simulink library "libc_control_pressure"  (R2015b)
settings: Solver=FixedStepDiscrete  StartTime=0.0  StopTime=Inf  FixedStep=0.004  RelTol=1e-3
PostLoadFcn:
  | , if any(exist('dsrtsu_mdlpostloadfcn', 'file') == [2, 3, 6]), try dsrtsu_mdlpostloadfcn('Execute', bdroot); catch fprintf('Error in PostLoadFcn (dsrtsu_mdlpostloadfcn) for model "%s":\n %s\n', bdroot, lasterr); end, end,
undefined symbols (not defined in the file or in its folder): CONST, den, DiscIntNeverNeededParam, num, p1i, tA
libraries: simulink x21, libc_parts_valves x17, libc_filters_diff x9, libbha_parts_bellows x4, libc_parts_tubes x2, PMC_lib x1
(part 2 of 2)

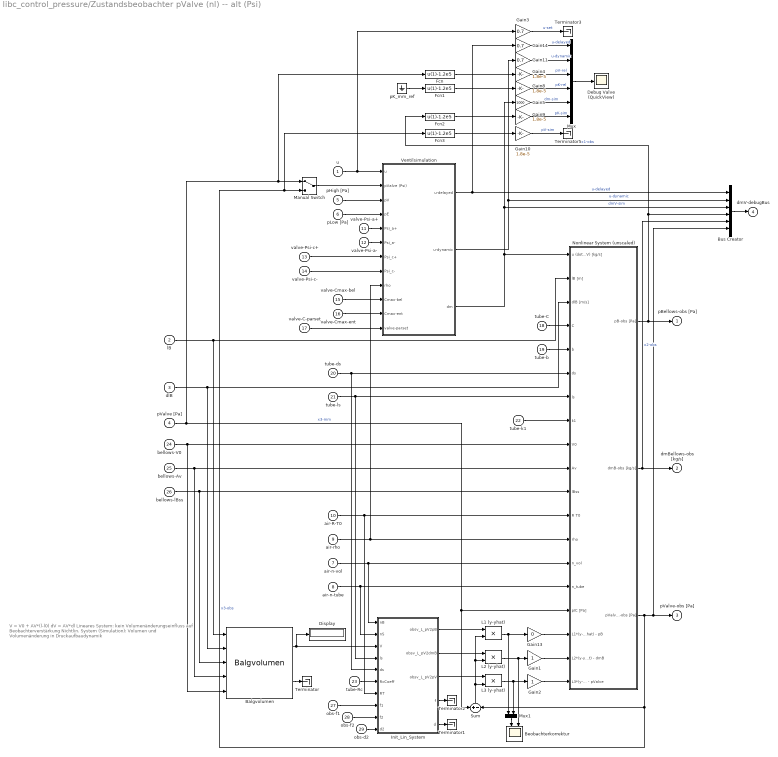
== system libc_control_pressure/Zustandsbeobachter pValve (nl) -- alt (Psi) ==
  note: V = V0 + AV*(l-l0)
      | dV = AV*dl
      |
      | Lineares System:
      | kein Volumenänderungseinfluss auf Beobachterverstärkung
      |
      | Nichtlin. System (Simulation):
      | Volumen und Volumenänderung in Druckaufbaudynamik
  u : Inport
  lB : Inport  Port=2
  dlB : Inport  Port=3
  pValve [Pa] : Inport  Port=4
  pHigh [Pa] : Inport  Port=5
  pLow [Pa] : Inport  Port=6
  air-n-vol : Inport  Port=7
  air-n-tube : Inport  Port=8
  air-rho : Inport  Port=9
  air-R-T0 : Inport  Port=10
  valve-Psi-a+ : Inport  Port=11
  valve-Psi-a- : Inport  Port=12
  valve-Psi-c+ : Inport  Port=13
  valve-Psi-c- : Inport  Port=14
  valve-Cmax-bel : Inport  Port=15
  valve-Cmax-ent : Inport  Port=16
  valve-C-parset : Inport  Port=17
  tube-C : Inport  Port=18
  tube-b : Inport  Port=19
  tube-ds : Inport  Port=20
  tube-ls : Inport  Port=21
  tube-k1 : Inport  Port=22
  tube-Rc : Inport  Port=23
  bellows-V0 : Inport  Port=24
  bellows-Av : Inport  Port=25
  bellows-lBss : Inport  Port=26
  obs-f1 : Inport  Port=27
  obs-f2 : Inport  Port=28
  obs-d2 : Inport  Port=29
  Balgvolumen : libbha_parts_bellows/Balgvolumen
  Beobachterkorrektur : Scope  NumInputPorts=2
  Bus Creator : BusCreator  Inputs=6
  Debug Valve (QuickView) : Scope
  Display : Display
  Fcn{,1..3} (4 alike) : Fcn  Expr=u(1)-1.2e5
  Gain1 : Gain
  Gain{4,8..10} (4 alike) : Gain  Gain=1.8e-5
  Gain11 : Gain  Gain=0.7
  Gain13 : Gain  Gain=0
  Gain14 : Gain  Gain=0.7
  Gain2 : Gain
  Gain3 : Gain  Gain=0.7
  Gain5 : Gain  Gain=1000
  Init_Lin_System : MATLAB Function  TreatAsAtomicUnit=on
  L1 (y-yhat) : Product
      settings: AttributesFormatString=sat: 0.1e5
  L2 (y-yhat) : Product
  L3 (y-yhat) : Product
  Manual Switch : ManualSwitch
  Mux : Mux  Inputs=6
  Mux1 : Mux  Inputs=2
  Nonlinear System (unscaled) : Subsystem
  Sum : Sum  Inputs=+|-
  Terminator{,1..3,5} (5 alike) : Terminator
  Ventilsimulation : Subsystem
  pK_mm_ref : Ground
  pBellows-obs [Pa] : Outport  PortDimensions=1
  dmBellows-obs [kg/s] : Outport  Port=2  PortDimensions=1
  pValve-obs [Pa] : Outport  Port=3  PortDimensions=1
  dmV-debugBus : Outport  Port=4
  wires:
  Gain14/1 -> Mux/1  "u-delayed"
  Ventilsimulation/2(u-dynamic) -> Gain11/1, Bus Creator/2  "u-dynamic"
  Gain13/1 -> Nonlinear System (unscaled)/17(L1*(y-yhat) - pB)
  Gain2/1 -> Nonlinear System (unscaled)/19(L3*(y-yhat) - pValve)
  Gain1/1 -> Nonlinear System (unscaled)/18(L2*(y-yhat) - dmB)
  Mux1/1 -> Beobachterkorrektur/1
  valve-Cmax-ent/1 -> Ventilsimulation/11(Cmax-ent)
  Gain11/1 -> Mux/2  "u-dynamic"
  Ventilsimulation/1(u-delayed) -> Gain14/1, Bus Creator/1  "u-delayed"
  Manual Switch/1 -> Ventilsimulation/2(pValve (Psi))
  Gain10/1 -> Terminator5/1  "pV-sim"
  Fcn3/1 -> Gain10/1
  Fcn2/1 -> Gain9/1
  Gain9/1 -> Mux/6  "pK-sim"
  Gain8/1 -> Mux/4  "pK-rel"
  Fcn1/1 -> Gain8/1
  pK_mm_ref/1 -> Fcn1/1
  Mux/1 -> Debug Valve (QuickView)/1
  Fcn/1 -> Gain4/1
  Gain5/1 -> Mux/5  "dm-sim"
  Gain4/1 -> Mux/3  "pV-rel"
  Gain3/1 -> Terminator3/1  "u-set"
  air-n-vol/1 -> Nonlinear System (unscaled)/14(n_vol), Init_Lin_System/1(nB)
  Ventilsimulation/3(dm) -> Nonlinear System (unscaled)/1(u (dotmV) [kg/s]), Gain5/1, Bus Creator/3  "dmV-sim"
  Init_Lin_System/4(f) -> Terminator2/1
  Init_Lin_System/5(d) -> Terminator1/1
  valve-Psi-c-/1 -> Ventilsimulation/8(Psi_c-)
  valve-Psi-c+/1 -> Ventilsimulation/7(Psi_c+)
  valve-Psi-a-/1 -> Ventilsimulation/6(Psi_a-)
  obs-f2/1 -> Init_Lin_System/9(f2)
  obs-d2/1 -> Init_Lin_System/10(d2)
  obs-f1/1 -> Init_Lin_System/8(f1)
  pLow [Pa]/1 -> Ventilsimulation/4(pE)
  pHigh [Pa]/1 -> Ventilsimulation/3(pV)
  valve-C-parset/1 -> Ventilsimulation/12(valve-parset)
  valve-Psi-a+/1 -> Ventilsimulation/5(Psi_a+)
  valve-Cmax-bel/1 -> Ventilsimulation/10(Cmax-bel)
  air-R-T0/1 -> Nonlinear System (unscaled)/12(R T0), Init_Lin_System/7(RT)
  air-rho/1 -> Ventilsimulation/9(rho), Nonlinear System (unscaled)/13(rho)
  u/1 -> Ventilsimulation/1(u), Gain3/1
  tube-Rc/1 -> Init_Lin_System/6(RcCoeff)
  bellows-Av/1 -> Nonlinear System (unscaled)/10(Av), Balgvolumen/4
  dlB/1 -> Nonlinear System (unscaled)/3(dlB [m/s]), Balgvolumen/2
  Balgvolumen/2 -> Terminator/1
  Balgvolumen/1 -> Init_Lin_System/3(V), Display/1
  tube-ls/1 -> Nonlinear System (unscaled)/7(ls), Init_Lin_System/4(ls)
  bellows-lBss/1 -> Nonlinear System (unscaled)/11(lBss), Balgvolumen/3
  bellows-V0/1 -> Nonlinear System (unscaled)/9(V0), Balgvolumen/5
  air-n-tube/1 -> Nonlinear System (unscaled)/15(n_tube), Init_Lin_System/2(nS)
  tube-k1/1 -> Nonlinear System (unscaled)/8(k1)
  lB/1 -> Nonlinear System (unscaled)/2(lB [m]), Balgvolumen/1
  tube-b/1 -> Nonlinear System (unscaled)/5(b)
  Init_Lin_System/1(obsv_L_pV2pB) -> L1 (y-yhat)/1
  Init_Lin_System/3(obsv_L_pV2pV) -> L3 (y-yhat)/1
  Init_Lin_System/2(obsv_L_pV2dmB) -> L2 (y-yhat)/1
  L3 (y-yhat)/1 -> Gain2/1, Mux1/2
  L2 (y-yhat)/1 -> Beobachterkorrektur/2, Gain1/1
  Nonlinear System (unscaled)/2(dmB-obs [kg/s]) -> dmBellows-obs [kg/s]/1, Bus Creator/5  "x2-obs"
  Nonlinear System (unscaled)/1(pB-obs [Pa]) -> pBellows-obs [Pa]/1, Bus Creator/4, Fcn2/1  "x1-obs"
  Nonlinear System (unscaled)/3(pValve-obs [Pa]) -> pValve-obs [Pa]/1, Bus Creator/6, Manual Switch/2, Fcn3/1, Sum/2  "x3-obs"
  Sum/1 -> L3 (y-yhat)/2, L2 (y-yhat)/2, L1 (y-yhat)/2
  L1 (y-yhat)/1 -> Gain13/1, Mux1/1
  pValve [Pa]/1 -> Manual Switch/1, Fcn/1, Nonlinear System (unscaled)/16(pIC [Pa]), Sum/1  "x3-mm"
  tube-C/1 -> Nonlinear System (unscaled)/4(C)
  tube-ds/1 -> Nonlinear System (unscaled)/6(ds), Init_Lin_System/5(ds)
  Bus Creator/1 -> dmV-debugBus/1

== system libc_control_pressure/Druckregler/Drucklinearsierung ==
  nu_in_PReg : Inport
  nu_in_Vorst : Inport  Port=2
  V : Inport  Port=3
  dV : Inport  Port=4
  p (E/A) : Inport  Port=5
  RT0 : Inport  Port=6
  nK : Inport  Port=7
  -Lf : Product  Inputs=*/**
  1/Lgx : Product  Inputs=//*
  mdot_soll : Product  Inputs=**
  nu-Lfx : Sum  Inputs=++|+
      settings: AttributesFormatString=|
      | früher ++-,
      | das ist aber falsch gewesen
  dm : Outport
  wires:
  p (E/A)/1 -> -Lf/4
  dV/1 -> -Lf/3
  -Lf/1 -> nu-Lfx/3
  mdot_soll/1 -> dm/1
  1/Lgx/1 -> mdot_soll/1
  nu-Lfx/1 -> mdot_soll/2
  nu_in_Vorst/1 -> nu-Lfx/2
  nu_in_PReg/1 -> nu-Lfx/1
  V/1 -> 1/Lgx/3, -Lf/2
  RT0/1 -> 1/Lgx/1
  nK/1 -> 1/Lgx/2, -Lf/1

== system libc_control_pressure/Druckregler/Folgeregler ==
  note: Vorsteuerung
  note: P-Regler
  p_soll : Inport
  dp_soll : Inport  Port=2
  p_ist : Inport  Port=3
  ctrl [ fgP enP enV ] : Inport  Port=4
  Demux : Demux  Outputs=3
  Product : Product
  Sw1 : Switch  Threshold=0.5
  Sw3 : Switch  Threshold=0.5
  null : Constant  Value=0
  null1 : Constant  Value=0
  omaga[rad/s] : Gain  Gain=2*pi
  reg_fehler : Sum  Inputs=+-
  e : Outport
  nu_P : Outport  Port=2
  nu_Vst : Outport  Port=3
  wires:
  Demux/1 -> omaga[rad/s]/1
  Product/1 -> Sw1/1
  null1/1 -> Sw1/3
  Demux/2 -> Sw1/2
  Demux/3 -> Sw3/2
  Sw1/1 -> nu_P/1
  Sw3/1 -> nu_Vst/1
  null/1 -> Sw3/3
  ctrl [ fgP enP enV ]/1 -> Demux/1
  dp_soll/1 -> Sw3/1
  reg_fehler/1 -> e/1, Product/1
  omaga[rad/s]/1 -> Product/2
  p_ist/1 -> reg_fehler/2
  p_soll/1 -> reg_fehler/1

== system libc_control_pressure/Ventilinvertierung FMText/Berechnung Ventilstellsignale mod-fav ==
  mp2_soll : Inport
  p2 : Inport  Port=2
  p1 : Inport  Port=3
  p0 : Inport  Port=4
  Ventilparam : Inport  Port=5  OutDataTypeStr=Bus: st_VentilParameter
  psi_min : Inport  Port=6
  kein_rueckstrom : Inport  Port=7
  BerechnungVentilstellsignale : Subsystem
      mask help: Umrechnung eines gewünschten Massenstroms in ein entsprechendes Ventilstellsignal.
  Bus Selector : BusSelector  OutputSignals=BP,BR
  Data Type Conversion : DataTypeConversion  OutDataTypeStr=double
  Product : Product
  Relational Operator : RelationalOperator  Operator=>  OutDataTypeStr=boolean
  Split_u : Subsystem
  Switch : Switch  Criteria=u2 > Threshold  Threshold=0.5
  Switch1 : Switch  Criteria=u2 > Threshold  Threshold=0.5
  Switch2 : Switch  Criteria=u2 > Threshold  Threshold=0.5
  inverse : Constant  Value=-1
  normal : Constant
  u : Outport
  wires:
  kein_rueckstrom/1 -> BerechnungVentilstellsignale/8(kein_rueckstrom)
  psi_min/1 -> BerechnungVentilstellsignale/7(psimin)
  Data Type Conversion/1 -> Switch/2, Switch1/2, Switch2/2
  Relational Operator/1 -> Data Type Conversion/1
  p0/1 -> Switch/3, Switch1/1, Relational Operator/2
  p1/1 -> Switch/1, Switch1/3, Relational Operator/1
  inverse/1 -> Switch2/3
  normal/1 -> Switch2/1
  Switch2/1 -> Product/1
  Product/1 -> Split_u/1(ut)
  BerechnungVentilstellsignale/1(ut) -> Product/2
  Switch1/1 -> BerechnungVentilstellsignale/4(p0_low)
  Switch/1 -> BerechnungVentilstellsignale/3(p1_high)
  Bus Selector/2 -> BerechnungVentilstellsignale/6(BR)  "<BR>"
  Bus Selector/1 -> BerechnungVentilstellsignale/5(BP)  "<BP>"
  Ventilparam/1 -> Bus Selector/1
  p2/1 -> BerechnungVentilstellsignale/2(p2_valve)
  mp2_soll/1 -> BerechnungVentilstellsignale/1(mp2_soll)
  Split_u/1(u) -> u/1

== system libc_control_pressure/Ventilinvertierung FMText/limit_p2 ==
  pV : Inport
  pH : Inport  Port=2
  pL : Inport  Port=3
  limit : Inport  Port=4
  Saturation Dynamic : simulink/Discontinuities/Saturation Dynamic  OutMin=[]  OutMax=[]  OutDataTypeStr=Inherit: Same as second input  OutDataType=fixdt(1, 16)  OutScaling=2^-10  DoSatur=off
  Sum : Sum  Inputs=|++
  Sum1 : Sum  Inputs=|+-
  dP [pA] : Constant  Value=0.1
  sw_p2s : Switch  Criteria=u2 > Threshold  Threshold=0.5
  pVlim : Outport
  wires:
  sw_p2s/1 -> pVlim/1
  pV/1 -> Saturation Dynamic/2, sw_p2s/3
  Saturation Dynamic/1 -> sw_p2s/1
  limit/1 -> sw_p2s/2
  Sum/1 -> Saturation Dynamic/3
  pL/1 -> Sum/1
  pH/1 -> Sum1/1
  Sum1/1 -> Saturation Dynamic/1
  dP [pA]/1 -> Sum/2, Sum1/2

== system libc_control_pressure/Ventilinvertierung FMText_simple/Berechnung Ventilstellsignale mod-fav ==
  mp2_soll : Inport
  p2 : Inport  Port=2
  p1 : Inport  Port=3
  p0 : Inport  Port=4
  Ventilparam : Inport  Port=5  OutDataTypeStr=Bus: st_VentilParameter
  psi_min : Inport  Port=6
  kein_rueckstrom : Inport  Port=7
  BerechnungVentilstellsignale : Subsystem
      mask help: Umrechnung eines gewünschten Massenstroms in ein entsprechendes Ventilstellsignal.
  Bus Selector : BusSelector  OutputSignals=BP,BR
  Data Type Conversion : DataTypeConversion  OutDataTypeStr=double
  Product : Product
  Relational Operator : RelationalOperator  Operator=>  OutDataTypeStr=boolean
  Split_u : Subsystem
  Switch : Switch  Criteria=u2 > Threshold  Threshold=0.5
  Switch1 : Switch  Criteria=u2 > Threshold  Threshold=0.5
  Switch2 : Switch  Criteria=u2 > Threshold  Threshold=0.5
  inverse : Constant  Value=-1
  normal : Constant
  u : Outport
  wires:
  Split_u/1(u) -> u/1
  mp2_soll/1 -> BerechnungVentilstellsignale/1(mp2_soll)
  p2/1 -> BerechnungVentilstellsignale/2(p2_valve)
  Ventilparam/1 -> Bus Selector/1
  Bus Selector/1 -> BerechnungVentilstellsignale/5(BP)  "<BP>"
  Bus Selector/2 -> BerechnungVentilstellsignale/6(BR)  "<BR>"
  Switch/1 -> BerechnungVentilstellsignale/3(p1_high)
  Switch1/1 -> BerechnungVentilstellsignale/4(p0_low)
  BerechnungVentilstellsignale/1(ut) -> Product/2
  Product/1 -> Split_u/1(ut)
  Switch2/1 -> Product/1
  normal/1 -> Switch2/1
  inverse/1 -> Switch2/3
  p1/1 -> Relational Operator/1, Switch1/3, Switch/1
  p0/1 -> Relational Operator/2, Switch1/1, Switch/3
  Relational Operator/1 -> Data Type Conversion/1
  Data Type Conversion/1 -> Switch2/2, Switch1/2, Switch/2
  psi_min/1 -> BerechnungVentilstellsignale/7(psimin)
  kein_rueckstrom/1 -> BerechnungVentilstellsignale/8(kein_rueckstrom)

== system libc_control_pressure/Ventilinvertierung FMText_simple/limit_p2 ==
  pV : Inport
  pH : Inport  Port=2
  pL : Inport  Port=3
  limit : Inport  Port=4
  Saturation Dynamic : simulink/Discontinuities/Saturation Dynamic  OutMin=[]  OutMax=[]  OutDataTypeStr=Inherit: Same as second input  OutDataType=fixdt(1, 16)  OutScaling=2^-10  DoSatur=off
  Sum : Sum  Inputs=|++
  Sum1 : Sum  Inputs=|+-
  dP [pA] : Constant  Value=0.1
  sw_p2s : Switch  Criteria=u2 > Threshold  Threshold=0.5
  pVlim : Outport
  wires:
  dP [pA]/1 -> Sum1/2, Sum/2
  Sum1/1 -> Saturation Dynamic/1
  pH/1 -> Sum1/1
  pL/1 -> Sum/1
  Sum/1 -> Saturation Dynamic/3
  limit/1 -> sw_p2s/2
  Saturation Dynamic/1 -> sw_p2s/1
  pV/1 -> sw_p2s/3, Saturation Dynamic/2
  sw_p2s/1 -> pVlim/1

== system libc_control_pressure/Ventilinvertierung MPYE/Psi Param ==
  b : Inport
  b-auto : MATLAB Function  TreatAsAtomicUnit=on
  a1 : Outport
  a2 : Outport  Port=2
  c0 : Outport  Port=3
  wires:
  b-auto/2(a2) -> a2/1
  b-auto/3(c0) -> c0/1
  b-auto/1(a1) -> a1/1
  b/1 -> b-auto/1(b)

== system libc_control_pressure/Zustandsbeobachter pValve (nl)/Nonlinear System (unscaled) ==
  u (dotmV) [kg/s] : Inport
  lB [m] : Inport  Port=2
  dlB [m/s] : Inport  Port=3
  C : Inport  Port=4
  b : Inport  Port=5
  ds : Inport  Port=6
  ls : Inport  Port=7
  k1 : Inport  Port=8
  V0 : Inport  Port=9
  Av : Inport  Port=10
  lBss : Inport  Port=11
  R T0 : Inport  Port=12
  rho : Inport  Port=13
  n_vol : Inport  Port=14
  n_tube : Inport  Port=15
  pIC [Pa] : Inport  Port=16
  L1*(y-yhat) - pB : Inport  Port=17
  L2*(y-yhat) - dmB : Inport  Port=18
  L3*(y-yhat) - pValve : Inport  Port=19
  Druckaufbau Balg : Subsystem
  Schlauchmodell 2. Ordnung (allg) : libc_parts_tubes/Schlauchmodell 2. Ordnung (allg)
  no_mf : Constant  Value=0
  pB-obs [Pa] : Outport
  dmB-obs [kg/s] : Outport  Port=2
  pValve-obs [Pa] : Outport  Port=3
  wires:
  n_vol/1 -> Druckaufbau Balg/5(n)
  Av/1 -> Druckaufbau Balg/8(Av)
  dlB [m/s]/1 -> Druckaufbau Balg/3(dlb [m/s])
  lBss/1 -> Druckaufbau Balg/7(lBss)
  V0/1 -> Druckaufbau Balg/9(V0)
  lB [m]/1 -> Druckaufbau Balg/2(lb [m])
  rho/1 -> Schlauchmodell 2. Ordnung (allg)/11
  R T0/1 -> Schlauchmodell 2. Ordnung (allg)/10, Druckaufbau Balg/6(RT0)
  b/1 -> Schlauchmodell 2. Ordnung (allg)/6
  u (dotmV) [kg/s]/1 -> Schlauchmodell 2. Ordnung (allg)/2
  pIC [Pa]/1 -> Druckaufbau Balg/1(pB_0), Schlauchmodell 2. Ordnung (allg)/3
  L3*(y-yhat) - pValve/1 -> Schlauchmodell 2. Ordnung (allg)/13
  L2*(y-yhat) - dmB/1 -> Schlauchmodell 2. Ordnung (allg)/14
  L1*(y-yhat) - pB/1 -> Druckaufbau Balg/10(L_pB)
  Schlauchmodell 2. Ordnung (allg)/2 -> pValve-obs [Pa]/1
  Druckaufbau Balg/1(p [Pa]) -> pB-obs [Pa]/1, Schlauchmodell 2. Ordnung (allg)/1
  Schlauchmodell 2. Ordnung (allg)/1 -> Druckaufbau Balg/4(mp [kg/s]), dmB-obs [kg/s]/1
  no_mf/1 -> Schlauchmodell 2. Ordnung (allg)/4
  C/1 -> Schlauchmodell 2. Ordnung (allg)/5
  ds/1 -> Schlauchmodell 2. Ordnung (allg)/7
  ls/1 -> Schlauchmodell 2. Ordnung (allg)/8
  n_tube/1 -> Schlauchmodell 2. Ordnung (allg)/12
  k1/1 -> Schlauchmodell 2. Ordnung (allg)/9

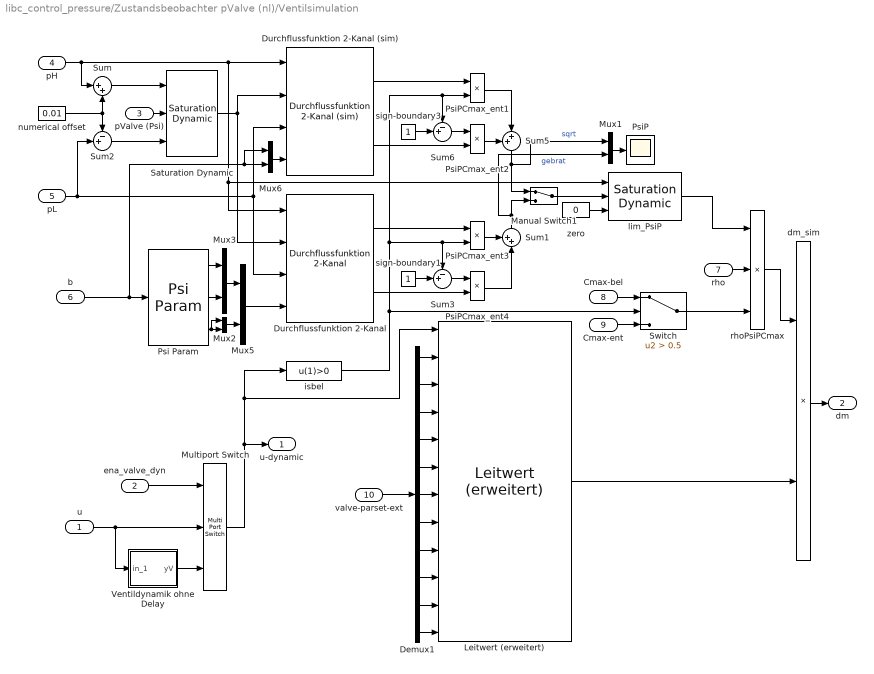
== system libc_control_pressure/Zustandsbeobachter pValve (nl)/Ventilsimulation ==
  u : Inport
  ena_valve_dyn : Inport  Port=2
  pValve (Psi) : Inport  Port=3
  pH : Inport  Port=4
  pL : Inport  Port=5
  b : Inport  Port=6
  rho : Inport  Port=7
  Cmax-bel : Inport  Port=8
  Cmax-ent : Inport  Port=9
  valve-parset-ext : Inport  Port=10
  Demux1 : Demux  Outputs=11
  Durchflussfunktion 2-Kanal : libc_parts_valves/Durchflussfunktion 2-Kanal
      settings: AttributesFormatString=gebrochenrational
  Durchflussfunktion 2-Kanal (sim) : libc_parts_valves/Durchflussfunktion 2-Kanal (sim)
      settings: AttributesFormatString=|
      | Wurzelfunktion
      | (nicht geeignet für Ventilinvertierung)
  Leitwert (erweitert) : libc_parts_valves/Leitwert (erweitert)  invertcomp=off
      settings: AttributesFormatString=|
      | inv: Cn --> u (on)
      | hin: u --> Cn (off)
      | Invertiert: %<invertcomp>
  Manual Switch1 : ManualSwitch
  Multiport Switch : MultiPortSwitch  DataPortOrder=Zero-based contiguous  Inputs=2
  Mux{1..3,5..6} (5 alike) : Mux  Inputs=2
  Psi Param : libc_parts_valves/Psi Param
      settings: AttributesFormatString=sqrt -> geb-rat
  PsiP : Scope
  PsiPCmax_ent{1..4} (4 alike) : Product
  Saturation Dynamic : simulink/Discontinuities/Saturation Dynamic  OutMin=[]  OutMax=[]  OutDataTypeStr=Inherit: Same as second input  OutDataType=fixdt(1, 16)  OutScaling=2^-10  DoSatur=off
  Sum : Sum  Inputs=|++
  Sum1 : Sum  Inputs=++|
  Sum2 : Sum  Inputs=-+|
  Sum3 : Sum  Inputs=-+|
  Sum5 : Sum  Inputs=++|
  Sum6 : Sum  Inputs=-+|
  Switch : Switch  Criteria=u2 > Threshold  Threshold=0.5
  Ventildynamik ohne Delay : Subsystem  mask(Ventilverzoegerung){wv=200*2*pi, dv=0.6, grenze=0.3, offset=0}
      mask prompts: wv "Eigenfreqenz"; dv "Daempfung"; grenze "Begrenzung"
      mask help: System 2. Ord. mit Begrenzung
      mask init:
      | [num,den]=ord2(wv,dv); t=0:0.5/wv:15/wv; u=0*t+1; u(1)=0;  y=lsim(num,den,u,t);
      mask Display: plot([0:0.1:1],[0 0.05 0.5 0.9 1.0 0.93 0.93 0.97 0.95 0.95 0.95]);
  dm_sim : Product  Inputs=**
  isbel : Fcn  Expr=u(1)>0
  lim_PsiP : simulink/Discontinuities/Saturation Dynamic  OutMin=[]  OutMax=[]  OutDataTypeStr=Inherit: Same as second input  OutDataType=fixdt(1, 16)  OutScaling=2^-10  DoSatur=off
      settings: AttributesFormatString=|
      | Unterer Schranke
      | im Entlüften nicht
      | pE sondern 0
  numerical offset : Constant  Value=0.01
  rhoPsiPCmax : Product  Inputs=***
  sign-boundary1 : Constant
  sign-boundary3 : Constant
  zero : Constant  Value=0
  u-dynamic : Outport
  dm : Outport  Port=2
  wires:
  dm_sim/1 -> dm/1
  Leitwert (erweitert)/1 -> dm_sim/2
  Demux1/1 -> Leitwert (erweitert)/2
  Demux1/2 -> Leitwert (erweitert)/3
  Demux1/5 -> Leitwert (erweitert)/6
  Demux1/6 -> Leitwert (erweitert)/7
  Demux1/3 -> Leitwert (erweitert)/4
  Demux1/4 -> Leitwert (erweitert)/5
  Demux1/7 -> Leitwert (erweitert)/8
  u/1 -> Multiport Switch/2, Ventildynamik ohne Delay/1(in_1)
  Multiport Switch/1 -> Leitwert (erweitert)/1, isbel/1, u-dynamic/1
  valve-parset-ext/1 -> Demux1/1
  Sum2/1 -> Saturation Dynamic/3
  numerical offset/1 -> Sum2/1, Sum/2
  pL/1 -> Sum2/2, Durchflussfunktion 2-Kanal (sim)/3, Durchflussfunktion 2-Kanal/3
  rhoPsiPCmax/1 -> dm_sim/1
  Saturation Dynamic/1 -> Durchflussfunktion 2-Kanal (sim)/2, Durchflussfunktion 2-Kanal/2
  pValve (Psi)/1 -> Saturation Dynamic/2
  lim_PsiP/1 -> rhoPsiPCmax/1
  Sum/1 -> Saturation Dynamic/1
  pH/1 -> Sum/1, Durchflussfunktion 2-Kanal (sim)/1, lim_PsiP/1, Durchflussfunktion 2-Kanal/1
  rho/1 -> rhoPsiPCmax/2
  Cmax-bel/1 -> Switch/1
  Ventildynamik ohne Delay/1(yV) -> Multiport Switch/3
  Switch/1 -> rhoPsiPCmax/3
  Cmax-ent/1 -> Switch/3
  zero/1 -> lim_PsiP/3
  ena_valve_dyn/1 -> Multiport Switch/1
  Demux1/9 -> Leitwert (erweitert)/10
  Demux1/10 -> Leitwert (erweitert)/11
  Demux1/8 -> Leitwert (erweitert)/9
  Demux1/11 -> Leitwert (erweitert)/12
  Mux1/1 -> PsiP/1
  Manual Switch1/1 -> lim_PsiP/2
  isbel/1 -> Switch/2, Sum3/1, PsiPCmax_ent3/2, Sum6/1, PsiPCmax_ent1/2
  b/1 -> Mux6/1, Mux6/2, Psi Param/1
  Mux5/1 -> Durchflussfunktion 2-Kanal/4
  Mux6/1 -> Durchflussfunktion 2-Kanal (sim)/4
  PsiPCmax_ent1/1 -> Sum5/2
  Durchflussfunktion 2-Kanal (sim)/1 -> PsiPCmax_ent1/1
  Durchflussfunktion 2-Kanal (sim)/2 -> PsiPCmax_ent2/2
  Sum6/1 -> PsiPCmax_ent2/1
  sign-boundary3/1 -> Sum6/2
  Durchflussfunktion 2-Kanal/1 -> PsiPCmax_ent3/1
  Durchflussfunktion 2-Kanal/2 -> PsiPCmax_ent4/2
  Sum3/1 -> PsiPCmax_ent4/1
  sign-boundary1/1 -> Sum3/2
  PsiPCmax_ent2/1 -> Sum5/1
  PsiPCmax_ent3/1 -> Sum1/1
  PsiPCmax_ent4/1 -> Sum1/2
  Sum1/1 -> Mux1/2, Manual Switch1/2  "gebrat"
  Sum5/1 -> Mux1/1, Manual Switch1/1  "sqrt"
  Psi Param/1 -> Mux3/1
  Psi Param/2 -> Mux3/2
  Psi Param/3 -> Mux2/1, Mux2/2
  Mux2/1 -> Mux5/2
  Mux3/1 -> Mux5/1

== system libc_control_pressure/Zustandsbeobachter pValve (nl) -- alt (Psi)/Nonlinear System (unscaled) ==
  u (dotmV) [kg/s] : Inport
  lB [m] : Inport  Port=2
  dlB [m/s] : Inport  Port=3
  C : Inport  Port=4
  b : Inport  Port=5
  ds : Inport  Port=6
  ls : Inport  Port=7
  k1 : Inport  Port=8
  V0 : Inport  Port=9
  Av : Inport  Port=10
  lBss : Inport  Port=11
  R T0 : Inport  Port=12
  rho : Inport  Port=13
  n_vol : Inport  Port=14
  n_tube : Inport  Port=15
  pIC [Pa] : Inport  Port=16
  L1*(y-yhat) - pB : Inport  Port=17
  L2*(y-yhat) - dmB : Inport  Port=18
  L3*(y-yhat) - pValve : Inport  Port=19
  Druckaufbau Balg : Subsystem
  Schlauchmodell 2. Ordnung (allg) : libc_parts_tubes/Schlauchmodell 2. Ordnung (allg)
  no_mf : Constant  Value=0
  pB-obs [Pa] : Outport
  dmB-obs [kg/s] : Outport  Port=2
  pValve-obs [Pa] : Outport  Port=3
  wires:
  n_vol/1 -> Druckaufbau Balg/5(n)
  Av/1 -> Druckaufbau Balg/8(Av)
  dlB [m/s]/1 -> Druckaufbau Balg/3(dlb [m/s])
  lBss/1 -> Druckaufbau Balg/7(lBss)
  V0/1 -> Druckaufbau Balg/9(V0)
  lB [m]/1 -> Druckaufbau Balg/2(lb [m])
  rho/1 -> Schlauchmodell 2. Ordnung (allg)/11
  R T0/1 -> Schlauchmodell 2. Ordnung (allg)/10, Druckaufbau Balg/6(RT0)
  b/1 -> Schlauchmodell 2. Ordnung (allg)/6
  u (dotmV) [kg/s]/1 -> Schlauchmodell 2. Ordnung (allg)/2
  pIC [Pa]/1 -> Druckaufbau Balg/1(pB_0), Schlauchmodell 2. Ordnung (allg)/3
  L3*(y-yhat) - pValve/1 -> Schlauchmodell 2. Ordnung (allg)/13
  L2*(y-yhat) - dmB/1 -> Schlauchmodell 2. Ordnung (allg)/14
  L1*(y-yhat) - pB/1 -> Druckaufbau Balg/10(L_pB)
  Schlauchmodell 2. Ordnung (allg)/2 -> pValve-obs [Pa]/1
  Druckaufbau Balg/1(p [Pa]) -> pB-obs [Pa]/1, Schlauchmodell 2. Ordnung (allg)/1
  Schlauchmodell 2. Ordnung (allg)/1 -> Druckaufbau Balg/4(mp [kg/s]), dmB-obs [kg/s]/1
  no_mf/1 -> Schlauchmodell 2. Ordnung (allg)/4
  C/1 -> Schlauchmodell 2. Ordnung (allg)/5
  ds/1 -> Schlauchmodell 2. Ordnung (allg)/7
  ls/1 -> Schlauchmodell 2. Ordnung (allg)/8
  n_tube/1 -> Schlauchmodell 2. Ordnung (allg)/12
  k1/1 -> Schlauchmodell 2. Ordnung (allg)/9

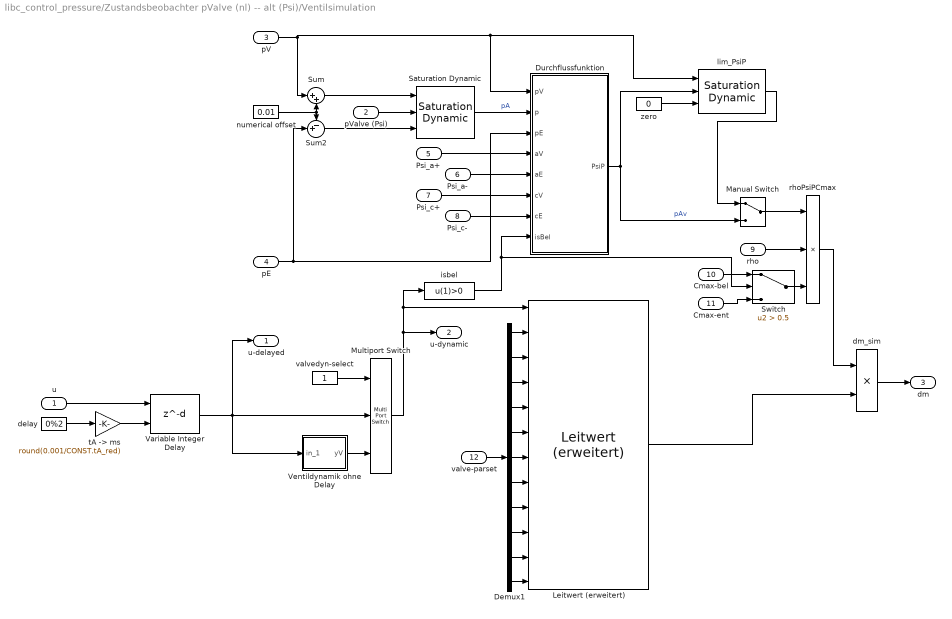
== system libc_control_pressure/Zustandsbeobachter pValve (nl) -- alt (Psi)/Ventilsimulation ==
  u : Inport
  pValve (Psi) : Inport  Port=2
  pV : Inport  Port=3
  pE : Inport  Port=4
  Psi_a+ : Inport  Port=5
  Psi_a- : Inport  Port=6
  Psi_c+ : Inport  Port=7
  Psi_c- : Inport  Port=8
  rho : Inport  Port=9
  Cmax-bel : Inport  Port=10
  Cmax-ent : Inport  Port=11
  valve-parset : Inport  Port=12
  Demux1 : Demux  Outputs=11
  Durchflussfunktion : MATLAB Function  TreatAsAtomicUnit=on
      settings: AttributesFormatString=saturated
  Leitwert (erweitert) : libc_parts_valves/Leitwert (erweitert)  invertcomp=off
      settings: AttributesFormatString=|
      | inv: Cn --> u (on)
      | hin: u --> Cn (off)
      | Invertiert: %<invertcomp>
  Manual Switch : ManualSwitch
  Multiport Switch : MultiPortSwitch  DataPortOrder=Zero-based contiguous  Inputs=2
  Saturation Dynamic : simulink/Discontinuities/Saturation Dynamic  OutMin=[]  OutMax=[]  OutDataTypeStr=Inherit: Same as second input  OutDataType=fixdt(1, 16)  OutScaling=2^-10  DoSatur=off
  Sum : Sum  Inputs=|++
  Sum2 : Sum  Inputs=-+|
  Switch : Switch  Criteria=u2 > Threshold  Threshold=0.5
  Variable Integer Delay : Delay  DelayLengthSource=Input port  DelayLength=0
      settings: AttributesFormatString=max delay %<DelayLengthUpperLimit>  InputPortMap=u0,p1
  Ventildynamik ohne Delay : Subsystem  mask(Ventilverzoegerung){wv=200*2*pi, dv=0.6, grenze=0.3, offset=0}
      mask prompts: wv "Eigenfreqenz"; dv "Daempfung"; grenze "Begrenzung"
      mask help: System 2. Ord. mit Begrenzung
      mask init:
      | [num,den]=ord2(wv,dv); t=0:0.5/wv:15/wv; u=0*t+1; u(1)=0;  y=lsim(num,den,u,t);
      mask Display: plot([0:0.1:1],[0 0.05 0.5 0.9 1.0 0.93 0.93 0.97 0.95 0.95 0.95]);
  delay : Constant  Value=0%2
      settings: AttributesFormatString=[ms] tA = 0.001
  dm_sim : Product  Inputs=**
  isbel : Fcn  Expr=u(1)>0
  lim_PsiP : simulink/Discontinuities/Saturation Dynamic  OutMin=[]  OutMax=[]  OutDataTypeStr=Inherit: Same as second input  OutDataType=fixdt(1, 16)  OutScaling=2^-10  DoSatur=off
      settings: AttributesFormatString=Unterer Schranke im Entlüften nicht pE sondern 0
  numerical offset : Constant  Value=0.01
  rhoPsiPCmax : Product  Inputs=***
  "tA -> ms" : Gain  Gain=round(0.001/CONST.tA_red)
  valvedyn-select : Constant
  zero : Constant  Value=0
  u-delayed : Outport
  u-dynamic : Outport  Port=2
  dm : Outport  Port=3
  wires:
  Demux1/11 -> Leitwert (erweitert)/12
  Demux1/10 -> Leitwert (erweitert)/11
  Demux1/9 -> Leitwert (erweitert)/10
  Demux1/8 -> Leitwert (erweitert)/9
  zero/1 -> lim_PsiP/3
  Cmax-ent/1 -> Switch/3
  Switch/1 -> rhoPsiPCmax/3
  "tA -> ms"/1 -> Variable Integer Delay/2
  delay/1 -> "tA -> ms"/1
  u/1 -> Variable Integer Delay/1
  valvedyn-select/1 -> Multiport Switch/1
  Ventildynamik ohne Delay/1(yV) -> Multiport Switch/3
  Psi_c-/1 -> Durchflussfunktion/7(cE)
  Psi_c+/1 -> Durchflussfunktion/6(cV)
  Psi_a-/1 -> Durchflussfunktion/5(aE)
  Cmax-bel/1 -> Switch/1
  rho/1 -> rhoPsiPCmax/2
  pV/1 -> lim_PsiP/1, Durchflussfunktion/1(pV), Sum/1
  Sum/1 -> Saturation Dynamic/1
  pValve (Psi)/1 -> Saturation Dynamic/2
  Saturation Dynamic/1 -> Durchflussfunktion/2(p)  "pA"
  Durchflussfunktion/1(PsiP) -> Manual Switch/2, lim_PsiP/2  "pAv"
  rhoPsiPCmax/1 -> dm_sim/1
  pE/1 -> Sum2/2, Durchflussfunktion/3(pE)
  numerical offset/1 -> Sum2/1, Sum/2
  Sum2/1 -> Saturation Dynamic/3
  Psi_a+/1 -> Durchflussfunktion/4(aV)
  valve-parset/1 -> Demux1/1
  Multiport Switch/1 -> isbel/1, Leitwert (erweitert)/1, u-dynamic/1
  Variable Integer Delay/1 -> Ventildynamik ohne Delay/1(in_1), Multiport Switch/2, u-delayed/1
  Demux1/7 -> Leitwert (erweitert)/8
  Demux1/4 -> Leitwert (erweitert)/5
  Demux1/3 -> Leitwert (erweitert)/4
  Demux1/6 -> Leitwert (erweitert)/7
  Demux1/5 -> Leitwert (erweitert)/6
  Demux1/2 -> Leitwert (erweitert)/3
  Demux1/1 -> Leitwert (erweitert)/2
  isbel/1 -> Durchflussfunktion/8(isBel), Switch/2
  Leitwert (erweitert)/1 -> dm_sim/2
  dm_sim/1 -> dm/1
  Manual Switch/1 -> rhoPsiPCmax/1
  lim_PsiP/1 -> Manual Switch/1

== system libc_control_pressure/Ventilinvertierung FMText/Berechnung Ventilstellsignale mod-fav/BerechnungVentilstellsignale ==
  mp2_soll : Inport
  p2_valve : Inport  Port=2
  p1_high : Inport  Port=3
  p0_low : Inport  Port=4
  BP : Inport  Port=5  OutDataTypeStr=Bus: st_Booster
  BR : Inport  Port=6  OutDataTypeStr=Bus: st_Booster
  psimin : Inport  Port=7
  kein_rueckstrom : Inport  Port=8
  Bus Selector : BusSelector  OutputSignals=C_max,b_max,b_min
  Bus Selector1 : BusSelector  OutputSignals=C_max,b_max,b_min
  Memory : Memory  InheritSampleTime=on
  Umrechnung Massenstrom in Ventilstellsignale : MATLAB Function
  ut : Outport
  wires:
  kein_rueckstrom/1 -> Umrechnung Massenstrom in Ventilstellsignale/12(kein_rueckstrom)
  psimin/1 -> Umrechnung Massenstrom in Ventilstellsignale/11(psimin)
  BR/1 -> Bus Selector1/1
  Bus Selector1/3 -> Umrechnung Massenstrom in Ventilstellsignale/10(bmin_ent)  "<b_min>"
  Bus Selector1/1 -> Umrechnung Massenstrom in Ventilstellsignale/8(C_ent)  "<C_max>"
  Bus Selector1/2 -> Umrechnung Massenstrom in Ventilstellsignale/9(b_ent)  "<b_max>"
  Bus Selector/2 -> Umrechnung Massenstrom in Ventilstellsignale/6(b_bel)  "<b_max>"
  Bus Selector/3 -> Umrechnung Massenstrom in Ventilstellsignale/7(bmin_bel)  "<b_min>"
  Bus Selector/1 -> Umrechnung Massenstrom in Ventilstellsignale/5(C_bel)  "<C_max>"
  BP/1 -> Bus Selector/1
  p1_high/1 -> Umrechnung Massenstrom in Ventilstellsignale/3(p1)
  p0_low/1 -> Umrechnung Massenstrom in Ventilstellsignale/4(p0)
  p2_valve/1 -> Umrechnung Massenstrom in Ventilstellsignale/2(p2)
  mp2_soll/1 -> Umrechnung Massenstrom in Ventilstellsignale/1(mp2)
  Memory/1 -> Umrechnung Massenstrom in Ventilstellsignale/13(ulast)
  Umrechnung Massenstrom in Ventilstellsignale/1(ut) -> Memory/1, ut/1

== system libc_control_pressure/Ventilinvertierung FMText/Berechnung Ventilstellsignale mod-fav/Split_u ==
  ut : Inport
  Gain : Gain  Gain=-1
  Mux : Mux  Inputs=2
  Saturation : Saturate  UpperLimit=1  LowerLimit=0
  Saturation1 : Saturate  UpperLimit=1  LowerLimit=0
  u : Outport
  wires:
  Saturation1/1 -> Mux/2
  Saturation/1 -> Mux/1
  Mux/1 -> u/1
  ut/1 -> Saturation/1, Gain/1
  Gain/1 -> Saturation1/1

== system libc_control_pressure/Ventilinvertierung FMText_simple/Berechnung Ventilstellsignale mod-fav/BerechnungVentilstellsignale ==
  mp2_soll : Inport
  p2_valve : Inport  Port=2
  p1_high : Inport  Port=3
  p0_low : Inport  Port=4
  BP : Inport  Port=5  OutDataTypeStr=Bus: st_Booster
  BR : Inport  Port=6  OutDataTypeStr=Bus: st_Booster
  psimin : Inport  Port=7
  kein_rueckstrom : Inport  Port=8
  Bus Selector : BusSelector  OutputSignals=C_max,b_max,b_min
  Bus Selector1 : BusSelector  OutputSignals=C_max,b_max,b_min
  Memory : Memory  InheritSampleTime=on
  Umrechnung Massenstrom in Ventilstellsignale : MATLAB Function
  ut : Outport
  wires:
  Umrechnung Massenstrom in Ventilstellsignale/1(ut) -> ut/1, Memory/1
  Memory/1 -> Umrechnung Massenstrom in Ventilstellsignale/13(ulast)
  mp2_soll/1 -> Umrechnung Massenstrom in Ventilstellsignale/1(mp2)
  p2_valve/1 -> Umrechnung Massenstrom in Ventilstellsignale/2(p2)
  p0_low/1 -> Umrechnung Massenstrom in Ventilstellsignale/4(p0)
  p1_high/1 -> Umrechnung Massenstrom in Ventilstellsignale/3(p1)
  BP/1 -> Bus Selector/1
  Bus Selector/1 -> Umrechnung Massenstrom in Ventilstellsignale/5(C_bel)  "<C_max>"
  Bus Selector/3 -> Umrechnung Massenstrom in Ventilstellsignale/7(bmin_bel)  "<b_min>"
  Bus Selector/2 -> Umrechnung Massenstrom in Ventilstellsignale/6(b_bel)  "<b_max>"
  Bus Selector1/2 -> Umrechnung Massenstrom in Ventilstellsignale/9(b_ent)  "<b_max>"
  Bus Selector1/1 -> Umrechnung Massenstrom in Ventilstellsignale/8(C_ent)  "<C_max>"
  Bus Selector1/3 -> Umrechnung Massenstrom in Ventilstellsignale/10(bmin_ent)  "<b_min>"
  BR/1 -> Bus Selector1/1
  psimin/1 -> Umrechnung Massenstrom in Ventilstellsignale/11(psimin)
  kein_rueckstrom/1 -> Umrechnung Massenstrom in Ventilstellsignale/12(kein_rueckstrom)

== system libc_control_pressure/Ventilinvertierung FMText_simple/Berechnung Ventilstellsignale mod-fav/Split_u ==
  ut : Inport
  Gain : Gain  Gain=-1
  Mux : Mux  Inputs=2
  Saturation : Saturate  UpperLimit=1  LowerLimit=0
  Saturation1 : Saturate  UpperLimit=1  LowerLimit=0
  u : Outport
  wires:
  Gain/1 -> Saturation1/1
  ut/1 -> Gain/1, Saturation/1
  Mux/1 -> u/1
  Saturation/1 -> Mux/1
  Saturation1/1 -> Mux/2

== system libc_control_pressure/Zustandsbeobachter pValve (nl)/Nonlinear System (unscaled)/Druckaufbau Balg ==
  pB_0 : Inport
  lb [m] : Inport  Port=2
  dlb [m/s] : Inport  Port=3
  mp [kg/s] : Inport  Port=4
  n : Inport  Port=5
  RT0 : Inport  Port=6
  lBss : Inport  Port=7
  Av : Inport  Port=8
  V0 : Inport  Port=9
  L_pB : Inport  Port=10
  Discrete-Time Integrator : DiscreteIntegrator  InitialConditionSource=external  InitialCondition=p1i  SampleTime=-1  ICPrevOutput=DiscIntNeverNeededParam  ICPrevScaledInput=DiscIntNeverNeededParam
  Druckdynamik (allg) : libbha_parts_bellows/Druckdynamik (allg)
  Sum1 : Sum  Inputs=|++
  p [Pa] : Outport  InitialOutput=0
  wires:
  V0/1 -> Druckdynamik (allg)/7
  Av/1 -> Druckdynamik (allg)/5
  lBss/1 -> Druckdynamik (allg)/6
  RT0/1 -> Druckdynamik (allg)/9
  lb [m]/1 -> Druckdynamik (allg)/1
  dlb [m/s]/1 -> Druckdynamik (allg)/2
  L_pB/1 -> Sum1/2
  pB_0/1 -> Discrete-Time Integrator/2
  Sum1/1 -> Discrete-Time Integrator/1
  Discrete-Time Integrator/1 -> p [Pa]/1, Druckdynamik (allg)/3
  mp [kg/s]/1 -> Druckdynamik (allg)/4
  Druckdynamik (allg)/1 -> Sum1/1
  n/1 -> Druckdynamik (allg)/8

== system libc_control_pressure/Zustandsbeobachter pValve (nl)/Ventilsimulation/Ventildynamik ohne Delay ==
  in_1 : Inport
  Saturation : Saturate  UpperLimit=grenze  LowerLimit=-grenze
  Sum : Sum  Inputs=+-  SaturateOnIntegerOverflow=on  InputSameDT=on  OutDataTypeStr=Inherit: Same as first input
  Sum2 : Sum  SaturateOnIntegerOverflow=on  InputSameDT=on  OutDataTypeStr=Inherit: Same as first input
  discrete filter : DiscreteTransferFcn  Numerator=num  Denominator=den  SampleTime=TS  mask{wv=wv, dv=dv, TS=CONST.tA_red}
      mask prompts: wv "Grenzfrequenz (rad/s)"; dv "Dämpfung"; TS "Sample Time"
      mask init:
      | csys = tf(wv^2,[1,2*dv*wv,0]);
      | [nums,dens] = tfdata(csys,'v');
      | [num,den] = tfdata(c2d(csys,TS),'v');
      settings: AttributesFormatString=w²/(s² + 2dws)
      mask Display: dpoly(nums,dens)
  p0 : Constant  Value=offset
  yV : Outport  InitialOutput=0
  wires:
  Sum2/1 -> yV/1
  in_1/1 -> Sum/1
  p0/1 -> Sum2/1
  discrete filter/1 -> Sum2/2, Sum/2
  Saturation/1 -> discrete filter/1
  Sum/1 -> Saturation/1

== system libc_control_pressure/Zustandsbeobachter pValve (nl) -- alt (Psi)/Nonlinear System (unscaled)/Druckaufbau Balg ==
  pB_0 : Inport
  lb [m] : Inport  Port=2
  dlb [m/s] : Inport  Port=3
  mp [kg/s] : Inport  Port=4
  n : Inport  Port=5
  RT0 : Inport  Port=6
  lBss : Inport  Port=7
  Av : Inport  Port=8
  V0 : Inport  Port=9
  L_pB : Inport  Port=10
  Discrete-Time Integrator : DiscreteIntegrator  InitialConditionSource=external  InitialCondition=p1i  SampleTime=-1  ICPrevOutput=DiscIntNeverNeededParam  ICPrevScaledInput=DiscIntNeverNeededParam
  Druckdynamik (allg) : libbha_parts_bellows/Druckdynamik (allg)
  Sum1 : Sum  Inputs=|++
  p [Pa] : Outport  InitialOutput=0
  wires:
  V0/1 -> Druckdynamik (allg)/7
  Av/1 -> Druckdynamik (allg)/5
  lBss/1 -> Druckdynamik (allg)/6
  RT0/1 -> Druckdynamik (allg)/9
  lb [m]/1 -> Druckdynamik (allg)/1
  dlb [m/s]/1 -> Druckdynamik (allg)/2
  L_pB/1 -> Sum1/2
  pB_0/1 -> Discrete-Time Integrator/2
  Sum1/1 -> Discrete-Time Integrator/1
  Discrete-Time Integrator/1 -> p [Pa]/1, Druckdynamik (allg)/3
  mp [kg/s]/1 -> Druckdynamik (allg)/4
  Druckdynamik (allg)/1 -> Sum1/1
  n/1 -> Druckdynamik (allg)/8

== system libc_control_pressure/Zustandsbeobachter pValve (nl) -- alt (Psi)/Ventilsimulation/Ventildynamik ohne Delay ==
  in_1 : Inport
  Saturation : Saturate  UpperLimit=grenze  LowerLimit=-grenze
  Sum : Sum  Inputs=+-  SaturateOnIntegerOverflow=on  InputSameDT=on  OutDataTypeStr=Inherit: Same as first input
  Sum2 : Sum  SaturateOnIntegerOverflow=on  InputSameDT=on  OutDataTypeStr=Inherit: Same as first input
  discrete filter : DiscreteTransferFcn  Numerator=num  Denominator=den  SampleTime=TS  mask{wv=wv, dv=dv, TS=CONST.tA_red}
      mask prompts: wv "Grenzfrequenz (rad/s)"; dv "Dämpfung"; TS "Sample Time"
      mask init:
      | csys = tf(wv^2,[1,2*dv*wv,0]);
      | [nums,dens] = tfdata(csys,'v');
      | [num,den] = tfdata(c2d(csys,TS),'v');
      settings: AttributesFormatString=w²/(s² + 2dws)
      mask Display: dpoly(nums,dens)
  p0 : Constant  Value=offset
  yV : Outport  InitialOutput=0
  wires:
  Sum/1 -> Saturation/1
  Saturation/1 -> discrete filter/1
  discrete filter/1 -> Sum/2, Sum2/2
  p0/1 -> Sum2/1
  in_1/1 -> Sum/1
  Sum2/1 -> yV/1

== matlab function libc_control_pressure/Ventilinvertierung FMText_simple/Berechnung Ventilstellsignale mod-fav/BerechnungVentilstellsignale/Umrechnung Massenstrom in Ventilstellsignale ==
  data: mp2 input; p2 input; p1 input; p0 input; ut output; C_bel input; b_bel input; bmin_bel input; C_ent input; b_ent input; bmin_ent input; psimin input; kein_rueckstrom input; ulast input
%%%%%%%%%%%%%%%%%%%%%%%%%%%%%%%%%%%%%%%%%%%%%%%%%%%%%%%%%%%%%%%%
%%%%   Umrechnung der Massenstroeme auf Ventilstellsignale   %%%%
%%%%%%%%%%%%%%%%%%%%%%%%%%%%%%%%%%%%%%%%%%%%%%%%%%%%%%%%%%%%%%%%
function ut  = mp2v(mp2,p2,p1,p0,C_bel,b_bel,bmin_bel,C_ent,b_ent,bmin_ent,psimin,kein_rueckstrom,ulast)
    % Uebergabe der Parameter  
    rho0 = 1.189;
    pss = 0.999;
    
    v = mp2;
    
    if(ulast<-1)
        ulast = -1;
    elseif(ulast>1)
        ulast = 1;
    end
    
    index = 0;
    
    if(v>0)
        p1t = p1;
        if kein_rueckstrom % p2 immer <= p1 !
            p2t = min(p1,p2);
        else
            p2t = p2;
        end
        
        % b-Wert Berechnung auf Basis des Stellsignals des letzten
        % Abtastzeitschritts:
        b = b_bel - ulast*(b_bel-bmin_bel);
        u = v/(C_bel * rho0 * psi(p1t, p2t, b, pss, psimin));
        
        % erneute Berechnung des b-Werts auf Basis des berechneten
        % Stellsignals
        uk1 = u;
        b = b_bel - u*(b_bel-bmin_bel);
        u = v/(C_bel * rho0 * psi(p1t, p2t, b, pss, psimin));
        
        % iterative Fortsetzung, solange die Stellsignalaenderung groesser als
        % der Schwellwert ist
        while(abs(u-uk1)>1e-4 && index<4)
            uk1 = u;
            b = b_bel - u*(b_bel-bmin_bel);
            u = v/(C_bel * rho0 * psi(p1t, p2t, b, pss, psimin));
            index = index + 1;
        end
    else
        p0t = p0;
        if kein_rueckstrom % p2 immer >= p0 !
            p2t = max(p0,p2);
        else
            p2t = p2;
        end
        
        % dito s.o.
        b = b_ent;
        u = -v/(C_ent * rho0 * psi(p0t, p2t, b, pss, psimin));
        
        uk1 = u;
        b = b_ent + u*(b_ent-bmin_ent);
        u = -v/(C_ent * rho0 * psi(p0t, p2t, b, pss, psimin));
        
        while(abs(u-uk1)>1e-4 && index<4)
            uk1 = u;
            b = b_ent + u*(b_ent-bmin_ent);
            u = -v/(C_ent * rho0 * psi(p0t, p2t, b, pss, psimin));
            index = index + 1;
        end
    end
    
    ut = u;
end

%%%%%%%%%%%%%%%%%%%%%%%%%%%%%%%%
%%%%   Durchflussfunktion   %%%%
%%%%%%%%%%%%%%%%%%%%%%%%%%%%%%%%
function ps_out = psi(p1_in, p2_in, b_val, pss, psimin)
    p1_in = abs(p1_in);
    p2_in = abs(p2_in);
    pH = max(p1_in,p2_in);
    pL = min(p1_in,p2_in);
    q = pL/pH;
    
    if(b_val>pss)
        b_val=pss;
    end
    
    y = sqrt(1.0-((pss-b_val)/(1-b_val))^2);
    dy = -(pss-b_val)/((1-b_val)^2)/sqrt(1-((pss-b_val)/(1-b_val))^2);
    apoly = -(pss*dy-y-dy)/(1+pss*pss-2*pss);
    bpoly = (pss*pss*dy-2*pss*y-pss*dy+y)/(1+pss*pss-2*pss);
    
    if (q < b_val)
        tmp = 1.0;
    elseif (q < pss)
        tmp = sqrt(1-((q-b_val)/(1-b_val))^2);
    else
        tmp = (1.0-q)*(apoly*q + bpoly);
    end
    
    if (pH == p1_in)
        vz = 1.0;
    else
        vz = -1.0;
    end
    
    ps_out = vz*pH*max(psimin,tmp);
end

== matlab function libc_control_pressure/Ventilinvertierung FMText/Berechnung Ventilstellsignale mod-fav/BerechnungVentilstellsignale/Umrechnung Massenstrom in Ventilstellsignale ==
  data: mp2 input; p2 input; p1 input; p0 input; ut output; C_bel input; b_bel input; bmin_bel input; C_ent input; b_ent input; bmin_ent input; psimin input; kein_rueckstrom input; ulast input
%%%%%%%%%%%%%%%%%%%%%%%%%%%%%%%%%%%%%%%%%%%%%%%%%%%%%%%%%%%%%%%%
%%%%   Umrechnung der Massenstroeme auf Ventilstellsignale   %%%%
%%%%%%%%%%%%%%%%%%%%%%%%%%%%%%%%%%%%%%%%%%%%%%%%%%%%%%%%%%%%%%%%
function ut  = mp2v(mp2,p2,p1,p0,C_bel,b_bel,bmin_bel,C_ent,b_ent,bmin_ent,psimin,kein_rueckstrom,ulast)
    % Uebergabe der Parameter  
    rho0 = 1.189;
    pss = 0.999;
    
    v = mp2;
    
    if(ulast<-1)
        ulast = -1;
    elseif(ulast>1)
        ulast = 1;
    end
    
    index = 0;
    
    if(v>0)
        p1t = p1;
        if kein_rueckstrom % p2 immer <= p1 !
            p2t = min(p1,p2);
        else
            p2t = p2;
        end
        
        % b-Wert Berechnung auf Basis des Stellsignals des letzten
        % Abtastzeitschritts:
        b = b_bel - ulast*(b_bel-bmin_bel);
        u = v/(C_bel * rho0 * psi(p1t, p2t, b, pss, psimin));
        
        % erneute Berechnung des b-Werts auf Basis des berechneten
        % Stellsignals
        uk1 = u;
        b = b_bel - u*(b_bel-bmin_bel);
        u = v/(C_bel * rho0 * psi(p1t, p2t, b, pss, psimin));
        
        % iterative Fortsetzung, solange die Stellsignalaenderung groesser als
        % der Schwellwert ist
        while(abs(u-uk1)>1e-4 && index<4)
            uk1 = u;
            b = b_bel - u*(b_bel-bmin_bel);
            u = v/(C_bel * rho0 * psi(p1t, p2t, b, pss, psimin));
            index = index + 1;
        end
    else
        p0t = p0;
        if kein_rueckstrom % p2 immer >= p0 !
            p2t = max(p0,p2);
        else
            p2t = p2;
        end
        
        % dito s.o.
        b = b_ent;
        u = -v/(C_ent * rho0 * psi(p0t, p2t, b, pss, psimin));
        
        uk1 = u;
        b = b_ent + u*(b_ent-bmin_ent);
        u = -v/(C_ent * rho0 * psi(p0t, p2t, b, pss, psimin));
        
        while(abs(u-uk1)>1e-4 && index<4)
            uk1 = u;
            b = b_ent + u*(b_ent-bmin_ent);
            u = -v/(C_ent * rho0 * psi(p0t, p2t, b, pss, psimin));
            index = index + 1;
        end
    end
    
    ut = u;
end

%%%%%%%%%%%%%%%%%%%%%%%%%%%%%%%%
%%%%   Durchflussfunktion   %%%%
%%%%%%%%%%%%%%%%%%%%%%%%%%%%%%%%
function ps_out = psi(p1_in, p2_in, b_val, pss, psimin)
    p1_in = abs(p1_in);
    p2_in = abs(p2_in);
    pH = max(p1_in,p2_in);
    pL = min(p1_in,p2_in);
    q = pL/pH;
    
    if(b_val>pss)
        b_val=pss;
    end
    
    y = sqrt(1.0-((pss-b_val)/(1-b_val))^2);
    dy = -(pss-b_val)/((1-b_val)^2)/sqrt(1-((pss-b_val)/(1-b_val))^2);
    apoly = -(pss*dy-y-dy)/(1+pss*pss-2*pss);
    bpoly = (pss*pss*dy-2*pss*y-pss*dy+y)/(1+pss*pss-2*pss);
    
    if (q < b_val)
        tmp = 1.0;
    elseif (q < pss)
        tmp = sqrt(1-((q-b_val)/(1-b_val))^2);
    else
        tmp = (1.0-q)*(apoly*q + bpoly);
    end
    
    if (pH == p1_in)
        vz = 1.0;
    else
        vz = -1.0;
    end
    
    ps_out = vz*pH*max(psimin,tmp);
end

== matlab function libc_control_pressure/Ventilinvertierung MPYE/Psi Param/b-auto ==
  data: b input; a1 output; a2 output; c0 output
function [a1,a2,c0]  = sqrt2gebrat(b)
%#codegen

    [a1,a2,c0] = psi_param(b);

end

== matlab function libc_control_pressure/Zustandsbeobachter pValve (nl)/Init_Lin_System ==
  data: nB input; nS input; V input; ls input; ds input; RcCoeff input; RT input; obsv_L_pV2pB output; f1 input; obsv_L_pV2dmB output; obsv_L_pV2pV output; f2 input; d2 input; f output; d output
function [obsv_L_pV2pB, obsv_L_pV2dmB, obsv_L_pV2pV, f, d] = obsgains(nB, nS, V, ls, ds, RcCoeff, RT, f1, f2, d2)
%#codegen

%CONST.tA = 0.001;
%BHASIM.tA = 0.0005;

%% Systemvariablen:

T = 1; % statt R und T wird nur R*T verwendet.
As = (ds/2)^2*pi;
Rc = RcCoeff*8*pi/As^2; % ?????
%RT0 = R*T;
    
%% Variablen-Skalierungen

scale_dm = 1e3;     % [kg/s]       [kg]->[ g]
scale_p  = 1e-5;    % [kg/m/s²]    [ m]->[nm]
if 1 % eigene Volumenskalierung
    scale_V  = 1e4; % [m³]         [ m]->[ l] = dm³ statt eigentlich nm³
    scale_ls = sqrt(scale_V*scale_p/scale_dm); 
    scale_As = sqrt(scale_V*scale_dm/scale_p);
else % Autoskalierung
    scale_V = (scale_dm/scale_p)^3;
    scale_ls = scale_dm/scale_p;
    scale_As = scale_dm^2/scale_p^2;
end
scale_R = scale_p*scale_V/scale_dm;
scale_Rc = scale_p/scale_dm;

nB = nB*1;              % [-]
nS = nS*1;              % [-]
T  = T*1;               % [K]
V  = V*scale_V;         % [m³]
RT = RT*scale_R;        % [Pa m³/kg/K = m²/s²/K]
ls = ls*scale_ls;       % [m]
As = As*scale_As;       % [m²]
Rc = Rc*scale_Rc;       % [1/m/s]

%% Analyse
% EV = -w(d+-sqrt(1-d²)
% --> w = sqrt(I²+R²), d = R/w

ev_real    = -(ls.*Rc)/2; 
ev_imag_sq = ((ls.*Rc).^2)/4 - pi^2/4*nS.*RT./ls.^2 - As./(ls.*V).*nB.*RT;

w = sqrt(ev_real.^2 + abs(ev_imag_sq));
d = -ev_real./w;
f = w/(2*pi);

%% Beobachterberechnung (Ackermann)
    
% Beobachter-Pole:

% if lambda is changed here, mm =/= ml
%lambda = [-w1*3; -w2*1.2*(d2-sqrt(1-d2^2)*1i); -w2*1.2*(d2+sqrt(1-d2^2)*1i)];

p00 =   (2*pi*f2).^2;
p01 = 2*(2*pi*f2).*d2;

p0 = p00.*(2*pi*f1);
p1 = p01.*(2*pi*f1) + p00;
p2 =      (2*pi*f1) + p01;

% Beobachter Ackermannformel für Ventildruck als Messgröße
%obsv_L_pV2pB  =                     4 .* ls .* n .^ (-1) .* pi .^ (-2) .* RT .^ (-1) .* T .^ (-1) .* V .^ (-1) .* (As .* n .* RT .* ((-1) .* p2 + ls .* Rc) .* T + p0 .* ls .* V); 
%obsv_L_pV2dmB = scale_p/scale_dm * (As .* ls .^ (-1) .* n .^ (-1) .* pi .^ (-2) .* RT .^ (-1) .* T .^ (-1) .* V .^ (-1) .* (4 .* As .* ls .* n .* RT .* T + ((-4) .* ls .^ 2 .* (p1 + ls .* Rc .* ((-1) .* p2 + ls .* Rc)) + n .* pi .^ 2 .* RT .* T) .* V));
%obsv_L_pV2pV  =                     p2 + (-1) .* ls .* Rc;

obsv_L_pV2pB  =                     4 .* ls .* nS .^ (-1) .* pi .^ (-2) .* RT .^ (-1) .* T .^ (-1) .* V .^ (-1) .* (As .* nB .* RT .* ((-1) .* p2 + ls .* Rc) .* T + p0 .* ls .* V);
obsv_L_pV2dmB = scale_p/scale_dm * (As .* ls .^ (-1) .* nS .^ (-1) .* pi .^ (-2) .* RT .^ (-1) .* T .^ (-1) .* V .^ (-1) .* (4 .* As .* ls .* nB .* RT .* T + ((-4) .* ls .^ 2 .* (p1 + ls .* Rc .* ((-1) .* p2 + ls .* Rc)) + nS .* pi .^ 2 .* RT .* T) .* V));
obsv_L_pV2pV  =                     p2 + (-1) .* ls .* Rc;

== matlab function libc_control_pressure/Zustandsbeobachter pValve (nl) -- alt (Psi)/Init_Lin_System ==
  data: nB input; nS input; V input; ls input; ds input; RcCoeff input; RT input; obsv_L_pV2pB output; f1 input; obsv_L_pV2dmB output; obsv_L_pV2pV output; f2 input; d2 input; f output; d output
function [obsv_L_pV2pB, obsv_L_pV2dmB, obsv_L_pV2pV, f, d] = obsgains(nB, nS, V, ls, ds, RcCoeff, RT, f1, f2, d2)
%#codegen

%CONST.tA = 0.001;
%BHASIM.tA = 0.0005;

%% Systemvariablen:

T = 1; % statt R und T wird nur R*T verwendet.
As = (ds/2)^2*pi;
Rc = RcCoeff*8*pi/As^2; % ?????
%RT0 = R*T;
    
%% Variablen-Skalierungen

scale_dm = 1e3;     % [kg/s]       [kg]->[ g]
scale_p  = 1e-5;    % [kg/m/s²]    [ m]->[nm]
if 1 % eigene Volumenskalierung
    scale_V  = 1e4; % [m³]         [ m]->[ l] = dm³ statt eigentlich nm³
    scale_ls = sqrt(scale_V*scale_p/scale_dm); 
    scale_As = sqrt(scale_V*scale_dm/scale_p);
else % Autoskalierung
    scale_V = (scale_dm/scale_p)^3;
    scale_ls = scale_dm/scale_p;
    scale_As = scale_dm^2/scale_p^2;
end
scale_R = scale_p*scale_V/scale_dm;
scale_Rc = scale_p/scale_dm;

nB = nB*1;              % [-]
nS = nS*1;              % [-]
T  = T*1;               % [K]
V  = V*scale_V;         % [m³]
RT = RT*scale_R;        % [Pa m³/kg/K = m²/s²/K]
ls = ls*scale_ls;       % [m]
As = As*scale_As;       % [m²]
Rc = Rc*scale_Rc;       % [1/m/s]

%% Analyse
% EV = -w(d+-sqrt(1-d²)
% --> w = sqrt(I²+R²), d = R/w

ev_real    = -(ls.*Rc)/2; 
ev_imag_sq = ((ls.*Rc).^2)/4 - pi^2/4*nS.*RT./ls.^2 - As./(ls.*V).*nB.*RT;

w = sqrt(ev_real.^2 + abs(ev_imag_sq));
d = -ev_real./w;
f = w/(2*pi);

%% Beobachterberechnung (Ackermann)
    
% Beobachter-Pole:

% if lambda is changed here, mm =/= ml
%lambda = [-w1*3; -w2*1.2*(d2-sqrt(1-d2^2)*1i); -w2*1.2*(d2+sqrt(1-d2^2)*1i)];

p00 =   (2*pi*f2).^2;
p01 = 2*(2*pi*f2).*d2;

p0 = p00.*(2*pi*f1);
p1 = p01.*(2*pi*f1) + p00;
p2 =      (2*pi*f1) + p01;

% Beobachter Ackermannformel für Ventildruck als Messgröße
%obsv_L_pV2pB  =                     4 .* ls .* n .^ (-1) .* pi .^ (-2) .* RT .^ (-1) .* T .^ (-1) .* V .^ (-1) .* (As .* n .* RT .* ((-1) .* p2 + ls .* Rc) .* T + p0 .* ls .* V); 
%obsv_L_pV2dmB = scale_p/scale_dm * (As .* ls .^ (-1) .* n .^ (-1) .* pi .^ (-2) .* RT .^ (-1) .* T .^ (-1) .* V .^ (-1) .* (4 .* As .* ls .* n .* RT .* T + ((-4) .* ls .^ 2 .* (p1 + ls .* Rc .* ((-1) .* p2 + ls .* Rc)) + n .* pi .^ 2 .* RT .* T) .* V));
%obsv_L_pV2pV  =                     p2 + (-1) .* ls .* Rc;

obsv_L_pV2pB  =                     4 .* ls .* nS .^ (-1) .* pi .^ (-2) .* RT .^ (-1) .* T .^ (-1) .* V .^ (-1) .* (As .* nB .* RT .* ((-1) .* p2 + ls .* Rc) .* T + p0 .* ls .* V);
obsv_L_pV2dmB = scale_p/scale_dm * (As .* ls .^ (-1) .* nS .^ (-1) .* pi .^ (-2) .* RT .^ (-1) .* T .^ (-1) .* V .^ (-1) .* (4 .* As .* ls .* nB .* RT .* T + ((-4) .* ls .^ 2 .* (p1 + ls .* Rc .* ((-1) .* p2 + ls .* Rc)) + nS .* pi .^ 2 .* RT .* T) .* V));
obsv_L_pV2pV  =                     p2 + (-1) .* ls .* Rc;

== matlab function libc_control_pressure/Zustandsbeobachter pValve (nl) -- alt (Psi)/Ventilsimulation/Durchflussfunktion ==
  data: pV input; p input; pE input; aV input; aE input; cV input; cE input; isBel input; PsiP output
function PsiP  = Psi_P(pV, p, pE, aV,aE,cV,cE, isBel)
%#codegen
    %aV = aVaEcVcE(1);
    %aE = aVaEcVcE(2);
    %cV = aVaEcVcE(3);
    %cE = aVaEcVcE(4);
    
    PsiP_bel = max(0,min(1,aV.*(pV-p)./(cV.*pV-p))) .* pV;
    PsiP_ent = max(0,min(1,aE.*(p-pE)./(cE.*p-pE))) .* p;

    PsiP = isBel.*PsiP_bel + (1-isBel).*PsiP_ent;
end
